simulink model "test2"  (R2017b)
settings: Solver=VariableStepAuto  StartTime=0.0  StopTime=10.0  RelTol=1e-3
values from neighbouring files (symbols this model uses):
  Cwy1 = 0.0074    [Parameters.m]
  Cwy2 = 0.0527    [Parameters.m]
  Cx = 52.92    [Parameters.m]
  Jyy = 0.78    [Parameters.m]
  k1_k = 0.2    [Parameters.m]
  k1_m = 5.09199    [Parameters.m]
  k2_k = 0.1    [Parameters.m]
  k2_m = 2.19    [Parameters.m]
  K_thruster = 2.89    [Parameters.m]
  kc = 57.2958    [Parameters.m]
  L = 1.760    (= 1.76)    [Parameters.m]
  lambda11 = 0.6    [Parameters.m]
  lambda55 = 0.9    [Parameters.m]
  m = 24.7    [Parameters.m]
  T_thruster = 0.1    [Parameters.m]
libraries: simulink x10, powerlib_meascontrol x1
settings Model: Creator=Eugene  LastModifiedBy=Eugene

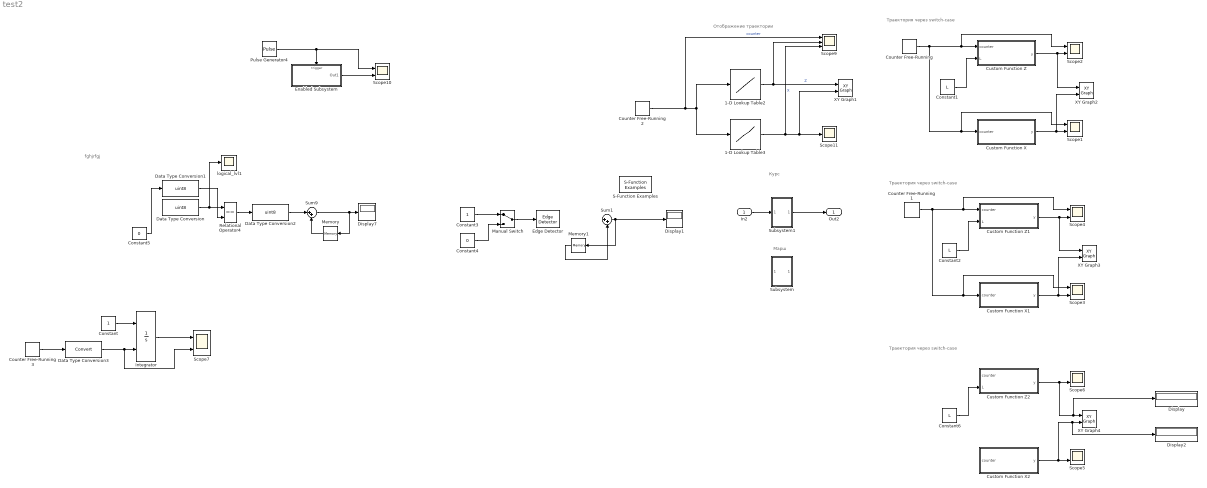
== system test2 ==
  note: Траектория через switch-case
  note: fghjrfgj
  note: Курс
  note: Марш
  note: Отображение траектории
  note: Траектория через switch-case
  note: Траектория через switch-case
  In2 : Inport
  1-D Lookup Table2 : Lookup_n-D  NumberOfTableDimensions=1  BreakpointsForDimension1=[0:7]  BreakpointsForDimension1FirstPoint=0  BreakpointsForDimension1DataTypeStr=uint8  Table=[0,0,L,L,2*L,2*L,3*L, 3*L]  TableDataTypeStr=double  InterpMethod=Flat  ExtrapMethod=Cubic spline  RemoveProtectionInput=on  InternalRulePriority=Speed  OutDataTypeStr=double  RndMeth=Zero  InputSameDT=on
  1-D Lookup Table3 : Lookup_n-D  NumberOfTableDimensions=1  BreakpointsForDimension1=[0:7]  BreakpointsForDimension1DataTypeStr=int16  Table=[0,25,25,0,0,25,25,0]  TableDataTypeStr=double  InterpMethod=Flat  RemoveProtectionInput=on  InternalRulePriority=Speed  OutDataTypeStr=double  RndMeth=Zero  InputSameDT=on
  Constant : Constant
  Constant1 : Constant  Value=L
  Constant2 : Constant  Value=L
  Constant3 : Constant
  Constant4 : Constant  Value=0
  Constant5 : Constant  Value=0
  Constant6 : Constant  Value=L
  Counter Free-Running : simulink/Sources/Counter Free-Running  NumBits=16  tsamp=-1
  Counter Free-Running1 : simulink/Sources/Counter Free-Running  NumBits=16  tsamp=-1
  Counter Free-Running2 : simulink/Sources/Counter Free-Running  NumBits=3  tsamp=1
  Counter Free-Running3 : simulink/Sources/Counter Free-Running  NumBits=3  tsamp=1
  Custom Function X : MATLAB Function  TreatAsAtomicUnit=on
  Custom Function X1 : MATLAB Function  TreatAsAtomicUnit=on
  Custom Function X2 : MATLAB Function  TreatAsAtomicUnit=on
  Custom Function Z : MATLAB Function  TreatAsAtomicUnit=on
  Custom Function Z1 : MATLAB Function  TreatAsAtomicUnit=on
  Custom Function Z2 : MATLAB Function  TreatAsAtomicUnit=on
  Data Type Conversion : DataTypeConversion  OutDataTypeStr=uint8
  Data Type Conversion1 : DataTypeConversion  OutDataTypeStr=uint8
  Data Type Conversion2 : DataTypeConversion  OutDataTypeStr=uint8
  Data Type Conversion3 : DataTypeConversion
  Display{,1..2,7} (4 alike) : Display
  Edge Detector : powerlib_meascontrol/Logic/Edge Detector  model=Falling  ic=0  Ts=0
      settings: SourceProductName=Simscape Power Systems  SourceProductBaseCode=PS
  Enabled Subsystem : Subsystem  TreatAsAtomicUnit=on
  Integrator : Integrator  ExternalReset=rising
  Manual Switch : ManualSwitch
  Memory : Memory
  Memory1 : Memory
  Pulse Generator4 : DiscretePulseGenerator  PulseType=Time based  PulseWidth=50
  Relational Operator4 : RelationalOperator  Operator===  OutDataTypeStr=boolean  RndMeth=Simplest
  S-Function Examples : simulink/User-Defined Functions/S-Function Examples
      settings: SourceProductName=Simulink  SourceProductBaseCode=SL
  Scope{1..7,10} (8 alike) : Scope  NumInputPorts=2
  Scope11 : Scope
  Scope9 : Scope  NumInputPorts=3
  Subsystem : Subsystem
  Subsystem1 : Subsystem
  Sum1 : Sum  Inputs=|++
  Sum9 : Sum  Inputs=|++
  XY Graph{1..4} (4 alike) : simulink/Sinks/XY Graph  xmin=-10  xmax=20  ymin=-10  ymax=30  st=-1
  logical_lvl1 : Scope
  Out2 : Outport
  wires:
  Subsystem1/1(Out2) -> Out2/1
  In2/1 -> Subsystem1/1(In2)
  Manual Switch/1 -> Edge Detector/1
  Constant3/1 -> Manual Switch/1
  Constant4/1 -> Manual Switch/2
  Memory1/1 -> Sum1/2
  Sum1/1 -> Display1/1, Memory1/1
  Enabled Subsystem/1(Out1) -> Scope10/2
  Pulse Generator4/1 -> Enabled Subsystem/Trigger, Scope10/1
  Constant5/1 -> Data Type Conversion1/1
  Data Type Conversion2/1 -> Sum9/1
  Data Type Conversion1/1 -> Relational Operator4/2
  Relational Operator4/1 -> Data Type Conversion2/1
  Data Type Conversion/1 -> logical_lvl1/1, Relational Operator4/1
  Memory/1 -> Sum9/2
  Sum9/1 -> Display7/1, Memory/1
  ? -> Data Type Conversion/1
  Counter Free-Running2/1 -> Scope9/1, 1-D Lookup Table2/1, 1-D Lookup Table3/1  "counter"
  1-D Lookup Table3/1 -> Scope11/1, XY Graph1/2, Scope9/3  "X"
  1-D Lookup Table2/1 -> XY Graph1/1, Scope9/2  "Z"
  Constant1/1 -> Custom Function Z/2(L)
  Counter Free-Running/1 -> Custom Function X/1(counter), Scope1/1, Scope2/1, Custom Function Z/1(counter)
  Custom Function X/1(y) -> Scope1/2, XY Graph2/2
  Custom Function Z/1(y) -> XY Graph2/1, Scope2/2
  Custom Function Z1/1(y) -> Scope4/2, XY Graph3/1
  Custom Function X1/1(y) -> XY Graph3/2, Scope3/2
  Counter Free-Running1/1 -> Custom Function Z1/1(counter), Scope4/1, Scope3/1, Custom Function X1/1(counter)
  Constant2/1 -> Custom Function Z1/2(L)
  Constant6/1 -> Custom Function Z2/2(L)
  ? -> Custom Function X2/1(counter), Scope5/1, Scope6/1, Custom Function Z2/1(counter)
  Custom Function X2/1(y) -> Scope5/2, Display2/1, XY Graph4/2
  Custom Function Z2/1(y) -> Display/1, XY Graph4/1, Scope6/2
  Constant/1 -> Integrator/1
  Counter Free-Running3/1 -> Data Type Conversion3/1
  Integrator/1 -> Scope7/1
  Data Type Conversion3/1 -> Scope7/2, Integrator/2

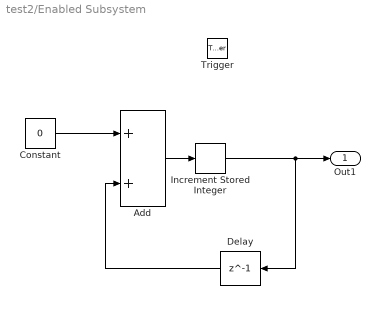
== system test2/Enabled Subsystem ==
  Trigger : TriggerPort  TriggerType=falling  VariantControl=Variant  PortDimensions=1
  Add : Sum
  Constant : Constant  Value=0
  Delay : Delay  DelayLength=1  InitialCondition=0
  Increment Stored Integer : simulink/Additional Math & Discrete/Additional Math: Increment - Decrement/Increment Stored Integer
      settings: SourceProductName=Simulink
  Out1 : Outport
  wires:
  Constant/1 -> Add/1
  Delay/1 -> Add/2
  Add/1 -> Increment Stored Integer/1
  Increment Stored Integer/1 -> Delay/1, Out1/1

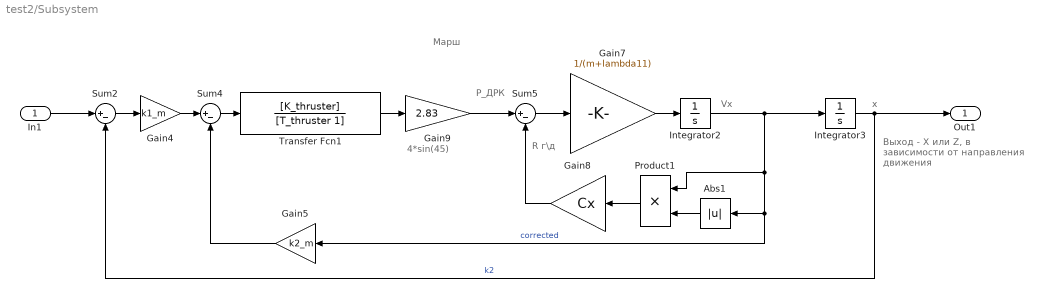
== system test2/Subsystem ==
  note: Выход - X или Z, в зависимости от направления движения
  note: 4*sin(45)
  note: R г\д
  note: x
  note: Vx
  note: P_ДРК
  note: Марш
  In1 : Inport
  Abs1 : Abs
  Gain4 : Gain  Gain=k1_m
  Gain5 : Gain  Gain=k2_m
  Gain7 : Gain  Gain=1/(m+lambda11)
  Gain8 : Gain  Gain=Cx
  Gain9 : Gain  Gain=2.83
  Integrator2 : Integrator
  Integrator3 : Integrator
  Product1 : Product
  Sum2 : Sum  Inputs=|+-
  Sum4 : Sum  Inputs=|+-
  Sum5 : Sum  Inputs=|+-
  Transfer Fcn1 : TransferFcn  Numerator=[K_thruster]  Denominator=[T_thruster 1]
  Out1 : Outport
  wires:
  In1/1 -> Sum2/1
  Sum2/1 -> Gain4/1
  Product1/1 -> Gain8/1
  Gain7/1 -> Integrator2/1
  Gain8/1 -> Sum5/2
  Integrator2/1 -> Integrator3/1, Gain5/1, Abs1/1, Product1/1  "corrected"
  Transfer Fcn1/1 -> Gain9/1
  Gain4/1 -> Sum4/1
  Sum4/1 -> Transfer Fcn1/1
  Integrator3/1 -> Out1/1, Sum2/2  "k2"
  Sum5/1 -> Gain7/1
  Gain9/1 -> Sum5/1
  Gain5/1 -> Sum4/2
  Abs1/1 -> Product1/2

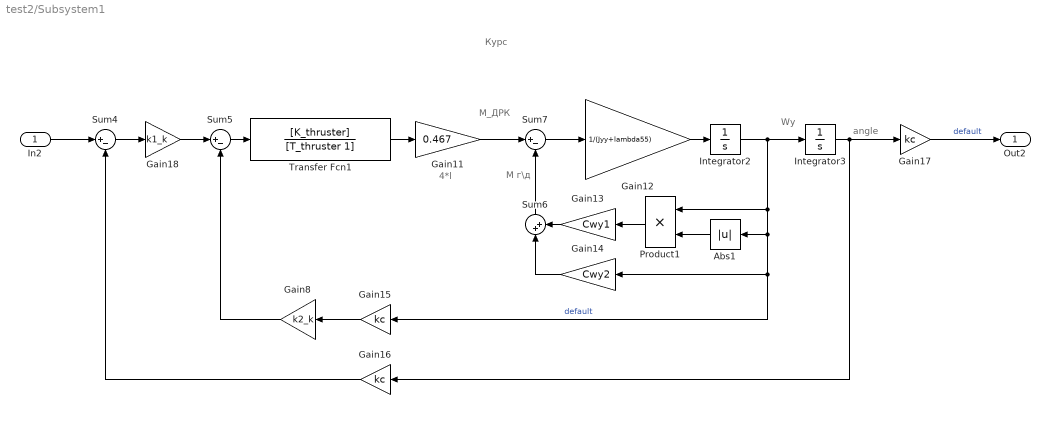
== system test2/Subsystem1 ==
  note: M г\д
  note: M_ДРК
  note: angle
  note: Wy
  note: 4*l
  note: Курс
  In2 : Inport
  Abs1 : Abs
  Gain11 : Gain  Gain=0.467
  Gain12 : Gain  Gain=1/(Jyy+lambda55)
  Gain13 : Gain  Gain=Cwy1
  Gain14 : Gain  Gain=Cwy2
  Gain15 : Gain  Gain=kc
  Gain16 : Gain  Gain=kc
  Gain17 : Gain  Gain=kc
  Gain18 : Gain  Gain=k1_k
  Gain8 : Gain  Gain=k2_k
  Integrator2 : Integrator
  Integrator3 : Integrator
  Product1 : Product
  Sum4 : Sum  Inputs=|+-
  Sum5 : Sum  Inputs=|+-
  Sum6 : Sum  Inputs=|++
  Sum7 : Sum  Inputs=|+-
  Transfer Fcn1 : TransferFcn  Numerator=[K_thruster]  Denominator=[T_thruster 1]
  Out2 : Outport
  wires:
  Integrator3/1 -> Gain17/1, Gain16/1
  Product1/1 -> Gain13/1
  Integrator2/1 -> Integrator3/1, Product1/1, Abs1/1, Gain14/1, Gain15/1  "default"
  Gain15/1 -> Gain8/1
  Gain18/1 -> Sum5/1
  Sum7/1 -> Gain12/1
  Gain16/1 -> Sum4/2
  Sum5/1 -> Transfer Fcn1/1
  Gain12/1 -> Integrator2/1
  Abs1/1 -> Product1/2
  Gain14/1 -> Sum6/1
  Sum4/1 -> Gain18/1
  Gain11/1 -> Sum7/1
  Gain13/1 -> Sum6/2
  Transfer Fcn1/1 -> Gain11/1
  Sum6/1 -> Sum7/2
  Gain8/1 -> Sum5/2
  Gain17/1 -> Out2/1  "default"
  In2/1 -> Sum4/1

== matlab function test2/Custom Function X ==
  data: counter input; y output
function y = fcn(counter)

%L = 1.76;

switch counter
    case 1
      y = 0;
    case 2
      y = 25;
    case 3
      y = 25;
    case 4
      y = 0;
    case 5
      y = 0;
    case 6
      y = 25;
    case 7
      y = 25;
    case 8
      y = 0;
    case 9
      y = 0;
    case 10
      y = 25;      
   otherwise
      y = 0;
end

== matlab function test2/Custom Function Z ==
  data: counter input; y output; L input
function y = fcn(counter, L)

%L = 1.76;

switch counter
    case 1
      y = 0;
    case 2
      y = 0;
    case 3
      y = L;
    case 4
      y = L;
    case 5
      y = 2*L;
    case 6
      y = 2*L;
    case 7
      y = 3*L;
    case 8
      y = 3*L;
    case 9
      y = 4*L;
    case 10
      y = 4*L;      
   otherwise
      y = 0;
end

== matlab function test2/Custom Function X1 ==
  data: counter input; y output
function y = fcn(counter)

%L = 1.76;

switch counter
    case 1
      y = 25;
    case 2
      y = 25;
    case 3
      y = 0;
    case 4
      y = 0;
    case 5
      y = 25;
    case 6
      y = 25;
    case 7
      y = 0;
    case 8
      y = 0;
    case 9
      y = 25;    
    case 10
      y = 25;
   otherwise
      y = 25;
end

== matlab function test2/Custom Function Z1 ==
  data: counter input; y output; L input
function y = fcn(counter, L)

%L = 1.76;

switch counter
    case 1
      y = 0;
    case 2
      y = L;
    case 3
      y = L;
    case 4
      y = 2*L;
    case 5
      y = 2*L;
    case 6
      y = 3*L;
    case 7
      y = 3*L;
    case 8
      y = 4*L;
    case 9
      y = 4*L;      
    case 10
      y = 5*L;      
   otherwise
      y = 0;
end

== matlab function test2/Custom Function X2 ==
  data: counter input; y output
function y = fcn(counter)

%L = 1.76;

switch counter
    case 1
      y = 25;
    case 2
      y = 25;
    case 3
      y = 0;
    case 4
      y = 0;
    case 5
      y = 25;
    case 6
      y = 25;
    case 7
      y = 0;
    case 8
      y = 0;
    case 9
      y = 25;    
    case 10
      y = 25;
   otherwise
      y = 25;
end

== matlab function test2/Custom Function Z2 ==
  data: counter input; y output; L input
function y = fcn(counter, L)

%L = 1.76;

switch counter
    case 1
      y = 0;
    case 2
      y = L;
    case 3
      y = L;
    case 4
      y = 2*L;
    case 5
      y = 2*L;
    case 6
      y = 3*L;
    case 7
      y = 3*L;
    case 8
      y = 4*L;
    case 9
      y = 4*L;      
    case 10
      y = 5*L;      
   otherwise
      y = 0;
end
